simulink model "esempio1_farrell_PI"  (R2025b)
settings: Solver=ode45  StartTime=0.0  StopTime=100  RelTol=1e-3  EnableMultiTasking=on
settings Model: Creator=Steph  LastModifiedBy=Steph
settings SolverCC: AlgebraicLoopSolver=TrustRegion
settings DataIOCC: LimitDataPoints=on  SaveFormat=Array  SignalLoggingSaveFormat=ModelDataLogs  ReturnWorkspaceOutputs=off
settings OptimizationCC: InitFltsAndDblsToZero=on  LifeSpan=inf
settings DebuggingCC: SaveWithParameterizedLinksMsg=none  UnderspecifiedInitializationDetection=Classic  MergeDetectMultiDrivingBlocksExec=none  SignalResolutionControl=TryResolveAllWithWarning  SolverPrmCheckMsg=warning  MultiTaskDSMMsg=warning  MultiTaskCondExecSysMsg=none  FcnCallInpInsideContextMsg=warning  UnconnectedInputMsg=warning  UnconnectedOutputMsg=warning  UnconnectedLineMsg=warning  SFUnexpectedBacktrackingDiag=warning  SFNoUnconditionalDefaultTransitionDiag=warning  SFExecutionAtInitializationDiag=none  ArithmeticOperatorsInVariantConditions=warning
settings HardwareCC: ProdBitPerPointer=32.0  ProdBitPerSizeT=32.0  ProdBitPerPtrDiffT=32.0  ProdLargestAtomicFloat=None  ProdIntDivRoundTo=Undefined  ProdEndianess=Unspecified  ProdWordSize=32.0  ProdHWDeviceType=32-bit Generic
settings ModelReferenceCC: PropagateSignalLabelsOutOfModel=off
settings RTWCC: GPUComputeCapability=3.5
settings CodeAppCC: StateflowObjectComments=on
settings GRTTargetCC: TargetFcnLib=ansi_tfl_tmw.mat  TargetLangStandard=C89/C90 (ANSI)  CombineOutputUpdateFcns=off  GRTInterface=on
settings ConfigComp: CovMetricSettings=dw  CovSaveCumulativeToWorkspaceVar=on  CovSaveSingleToWorkspaceVar=on

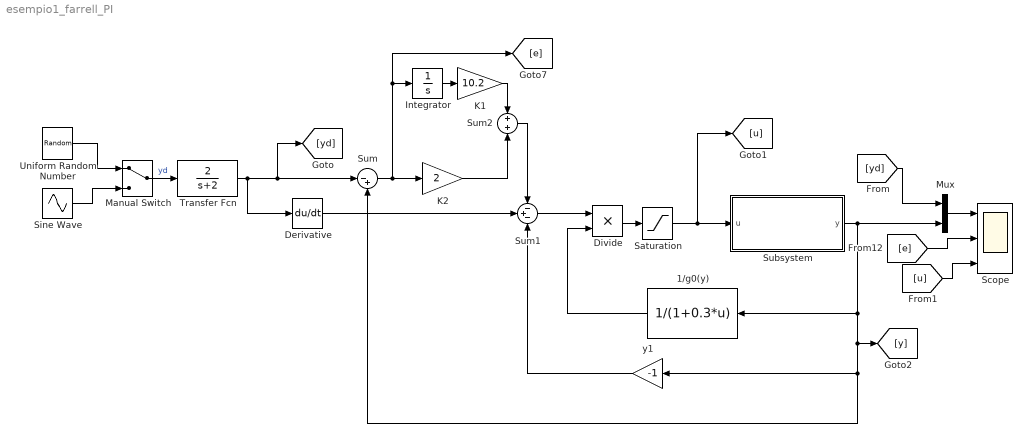
== system esempio1_farrell_PI ==
  1/g0(y) : Fcn  Expr=1/(1+0.3*u)
  Derivative : Derivative
  Divide : Product  Inputs=**
  Integrator : Integrator
  K1 : Gain  Gain=10.2
  K2 : Gain  Gain=2
  Manual Switch : ManualSwitch
  Mux : Mux  Inputs=2
  Saturation : Saturate  UpperLimit=10  LowerLimit=-10
  Scope : Scope  NumInputPorts=3
      settings: TimeSpan=100  ActiveDisplayYMinimum=-7.0047853797915387  ActiveDisplayYMaximum=84.564171108734257
  Sine Wave : Sin  Amplitude=20  Bias=40  SampleTime=0
  Subsystem : Subsystem
  Sum : Sum  Inputs=|-+
  Sum1 : Sum  Inputs=-+-
  Sum2 : Sum
  Transfer Fcn : TransferFcn  Numerator=[2]  Denominator=[1 2]
  Uniform Random Number : UniformRandomNumber  Minimum=20  Maximum=60  SampleTime=10
  y1 : Gain  Gain=-1
  wires:
  Subsystem/1(y) -> Mux/2, [y], Sum/2, y1/1, 1/g0(y)/1
  Sum/1 -> K2/1, Integrator/1, [e]
  Derivative/1 -> Sum1/2
  [yd] -> Mux/1
  Mux/1 -> Scope/1
  Sum1/1 -> Divide/1
  Divide/1 -> Saturation/1
  Manual Switch/1 -> Transfer Fcn/1  "yd"
  Uniform Random Number/1 -> Manual Switch/1
  Integrator/1 -> K1/1
  K2/1 -> Sum2/2
  Sum2/1 -> Sum1/1
  Saturation/1 -> Subsystem/1(u), [u]
  K1/1 -> Sum2/1
  Transfer Fcn/1 -> Derivative/1, Sum/1, [yd]
  [u] -> Scope/3
  [e] -> Scope/2
  Sine Wave/1 -> Manual Switch/2
  1/g0(y)/1 -> Divide/2
  y1/1 -> Sum1/3

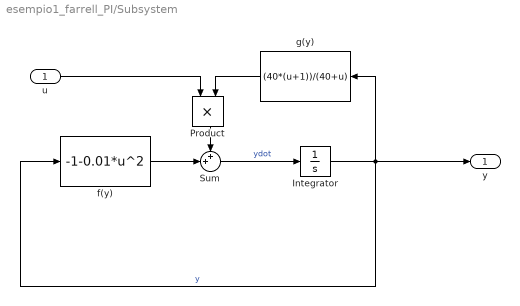
== system esempio1_farrell_PI/Subsystem ==
  u : Inport
  Integrator : Integrator
  Product : Product  RndMeth=Zero
  Sum : Sum  Inputs=++|
  f(y) : Fcn  Expr=-1-0.01*u^2
  g(y) : Fcn  Expr=(40*(u+1))/(40+u)
  y : Outport
  wires:
  Sum/1 -> Integrator/1  "ydot"
  f(y)/1 -> Sum/2
  Product/1 -> Sum/1
  g(y)/1 -> Product/2
  u/1 -> Product/1
  Integrator/1 -> y/1, g(y)/1, f(y)/1  "y"
